simulink model "unidade3TestarBomba"  (R2015b)
settings: Solver=ode1  StartTime=0.0  StopTime=inf  FixedStep=0.002  RelTol=1e-3
PostLoadFcn:
  | qc_set_target_type(getConfigSet(bdroot, 'QUARC Default Target Configuration'));
undefined symbols (not defined in the file or in its folder): HIL
libraries: quarc_library x3
settings Model: SimulationMode=external  ExtModeTrigDuration=30000  Creator=MLevis  LastModifiedBy=UFRN
settings SolverCC: PositivePriorityOrder=on
settings DataIOCC: SaveFormat=Array  SignalLoggingSaveFormat=ModelDataLogs
settings OptimizationCC: ExpressionDepthLimit=2147483647  InitFltsAndDblsToZero=on
settings DebuggingCC: SaveWithParameterizedLinksMsg=none  UnderspecifiedInitializationDetection=Classic  MergeDetectMultiDrivingBlocksExec=none  SolverPrmCheckMsg=warning  MultiTaskDSMMsg=warning  MultiTaskCondExecSysMsg=none  FcnCallInpInsideContextMsg=UseLocalSettings  StateNameClashWarn=warning
settings HardwareCC: ProdBitPerPointer=32  ProdLargestAtomicFloat=None  ProdIntDivRoundTo=Undefined  ProdEndianess=Unspecified  ProdWordSize=32  ProdHWDeviceType=32-bit Generic
settings RTWCC: SystemTargetFile=quarc_win64.tlc  TemplateMakefile=quarc_default_tmf  Description=QUARC Win64 Target
settings GRTTargetCC: ParMdlRefBuildCompliant=off  CompOptLevelCompliant=off  GeneratePreprocessorConditionals=Disable all  CombineOutputUpdateFcns=off  MatFileLogging=off  GRTInterface=on  UseToolchainInfoCompliant=off  ExtMode=on  ExtModeMexFile=quarc_comm
settings ConfigComp: CovModelRefEnable=Off

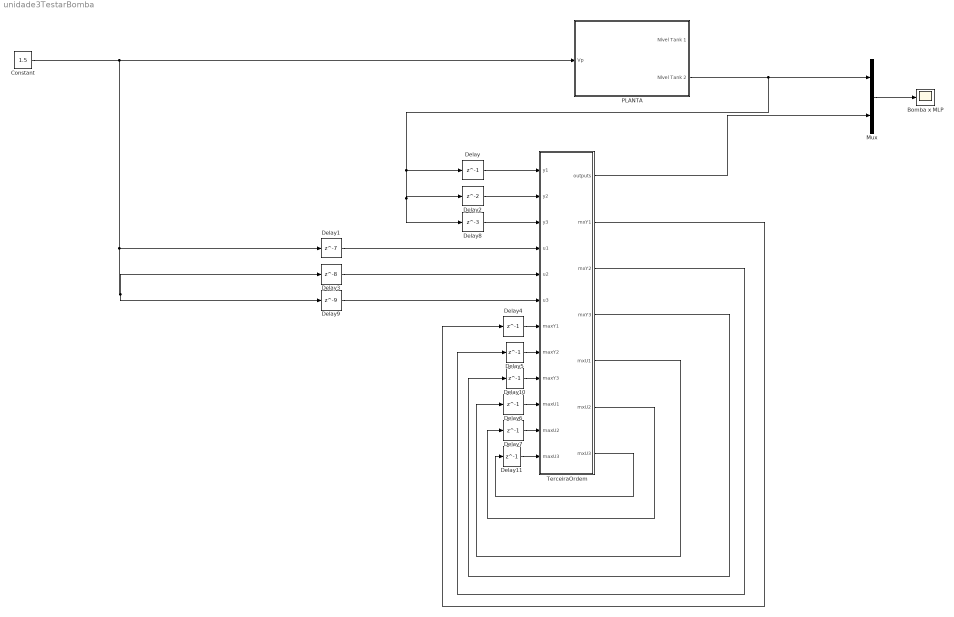
== system unidade3TestarBomba ==
  "Bomba x MLP " : Scope
  Constant : Constant  Value=1.5
  Delay{,4..7,10..11} (7 alike) : Delay  DelayLength=1  InitialCondition=0
  Delay1 : Delay  DelayLength=7  InitialCondition=0
  Delay2 : Delay  InitialCondition=0
  Delay3 : Delay  DelayLength=8  InitialCondition=0
  Delay8 : Delay  DelayLength=3  InitialCondition=0
  Delay9 : Delay  DelayLength=9  InitialCondition=0
  Mux : Mux  Inputs=2
  PLANTA : Subsystem
  "TerceiraOrdem " : MATLAB Function  TreatAsAtomicUnit=on
  wires:
  Mux/1 -> "Bomba x MLP "/1
  Delay/1 -> "TerceiraOrdem "/1(y1)
  Delay1/1 -> "TerceiraOrdem "/4(u1)
  Delay2/1 -> "TerceiraOrdem "/2(y2)
  Delay3/1 -> "TerceiraOrdem "/5(u2)
  PLANTA/2(Nível Tank 2) -> Delay2/1, Delay8/1, Delay/1, Mux/1
  Constant/1 -> Delay9/1, Delay3/1, Delay1/1, PLANTA/1(Vp)
  "TerceiraOrdem "/1(outputs) -> Mux/2
  "TerceiraOrdem "/2(mxY1) -> Delay4/1
  "TerceiraOrdem "/3(mxY2) -> Delay5/1
  Delay4/1 -> "TerceiraOrdem "/7(maxY1)
  Delay5/1 -> "TerceiraOrdem "/8(maxY2)
  Delay6/1 -> "TerceiraOrdem "/10(maxU1)
  Delay7/1 -> "TerceiraOrdem "/11(maxU2)
  Delay8/1 -> "TerceiraOrdem "/3(y3)
  Delay9/1 -> "TerceiraOrdem "/6(u3)
  Delay11/1 -> "TerceiraOrdem "/12(maxU3)
  Delay10/1 -> "TerceiraOrdem "/9(maxY3)
  "TerceiraOrdem "/4(mxY3) -> Delay10/1
  "TerceiraOrdem "/7(mxU3) -> Delay11/1
  "TerceiraOrdem "/6(mxU2) -> Delay7/1
  "TerceiraOrdem "/5(mxU1) -> Delay6/1

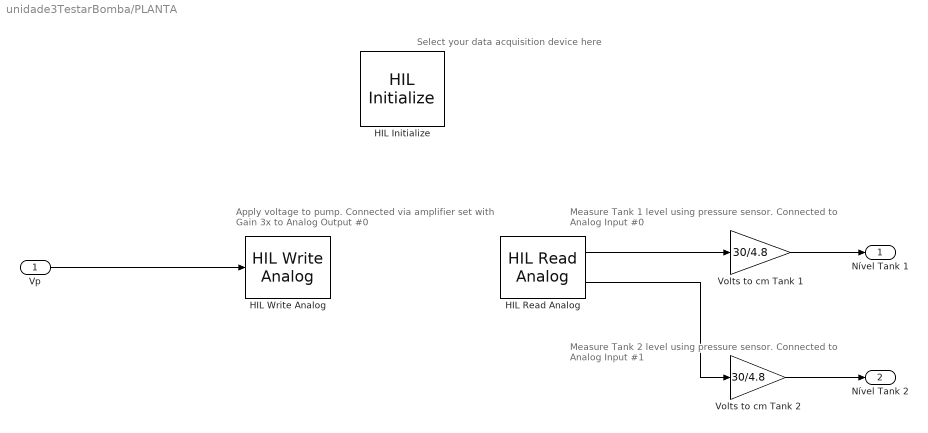
== system unidade3TestarBomba/PLANTA ==
  note: Select your data acquisition device here
  note: Apply voltage to pump.
      | Connected via amplifier set with Gain 3x
      | to  Analog Output #0
  note: Measure Tank 2 level using pressure sensor.
      | Connected to Analog Input #1
  note: Measure Tank 1 level using pressure sensor.
      | Connected to Analog Input #0
  Vp : Inport
  HIL Initialize : quarc_library/Data Acquisition/Generic/Configuration/HIL Initialize  object_name=HIL-1  board_type=q8_usb  board_number=0  board_options=update_rate=normal;decimation=1  exclusive=off  active=off  hardware_clocks=[0:2]  clock_modes=[]  initial_clock_frequencies=[]  set_clock_params_at_start=off  set_clock_params_at_switch_in=off  set_clock_frequencies_at_start=off  set_clock_frequencies_at_switch_in=off  analog_input_channels=[0:7]  analog_input_maximums=10  analog_input_minimums=-10  set_analog_input_params_at_start=on  set_analog_input_params_at_switch_in=off  analog_output_channels=[0:7]  analog_output_maximums=10  analog_output_minimums=-10  initial_analog_outputs=[0]  final_analog_outputs=[0]  watchdog_analog_outputs=0  set_analog_output_params_at_start=on  set_analog_output_params_at_switch_in=off  set_analog_outputs_at_start=on  set_analog_outputs_at_switch_in=off  set_analog_outputs_at_terminate=on  set_analog_outputs_at_switch_out=off  set_analog_outputs_on_watchdog=off  digital_input_channels=[]  digital_output_channels=[]  digital_output_configuration=[]  initial_digital_outputs=[1]  final_digital_outputs=[1]  watchdog_digital_outputs=[1]  set_digital_output_params_at_start=off  set_digital_output_params_at_switch_in=off  set_digital_outputs_at_start=on  set_digital_outputs_at_switch_in=off  set_digital_outputs_at_terminate=on  set_digital_outputs_at_switch_out=off  set_digital_outputs_on_watchdog=off  encoder_channels=[0:7]  quadrature=[4]  encoder_filter_frequency=[]  initial_encoder_counts=[0]  set_encoder_params_at_start=on  set_encoder_params_at_switch_in=off  set_encoder_counts_at_start=on  set_encoder_counts_at_switch_in=off  pwm_channels=[0:7]  pwm_modes=0  pwm_frequency=99.532799999999995e6/4095  pwm_configuration=[0]  pwm_alignment=[0]  pwm_polarity=[1]  pwm_leading_deadband=[0]  pwm_trailing_deadband=[0]  initial_pwm_outputs=[0]  final_pwm_outputs=[0]  watchdog_pwm_outputs=[0]  set_pwm_params_at_start=on  set_pwm_params_at_switch_in=off  set_pwm_outputs_at_start=on  set_pwm_outputs_at_switch_in=off  set_pwm_outputs_at_terminate=on  set_pwm_outputs_at_switch_out=off  set_pwm_outputs_on_watchdog=off  other_output_channels=[]  initial_other_outputs=[]  final_other_outputs=[]  watchdog_other_outputs=[]  set_other_outputs_at_start=off  set_other_outputs_at_switch_in=off  set_other_outputs_at_terminate=off  set_other_outputs_at_switch_out=off  set_other_outputs_on_watchdog=off
  HIL Read Analog : quarc_library/Data Acquisition/Generic/Immediate I//O/HIL Read Analog  object_name=HIL-1  channels=[0:1]  sample_time=qc_get_step_size  active=on  vector_output=off
  HIL Write Analog : quarc_library/Data Acquisition/Generic/Immediate I//O/HIL Write Analog  object_name=HIL-1  channels=0  sample_time=-1  active=off  vector_input=off
  "Volts to cm Tank 1 " : Gain  Gain=30/4.8
  Volts to cm Tank 2 : Gain  Gain=30/4.8
  Nível Tank 1 : Outport
  Nível Tank 2 : Outport  Port=2
  wires:
  HIL Read Analog/1 -> "Volts to cm Tank 1 "/1
  HIL Read Analog/2 -> Volts to cm Tank 2/1
  Vp/1 -> HIL Write Analog/1
  "Volts to cm Tank 1 "/1 -> Nível Tank 1/1
  Volts to cm Tank 2/1 -> Nível Tank 2/1

== matlab function unidade3TestarBomba/TerceiraOrdem  ==
  data: y1 input; y2 input; y3 input; u1 input; outputs output; u2 input; u3 input; maxY1 input; maxY2 input; maxY3 input; maxU1 input; maxU2 input; mxY1 output; mxY2 output; mxY3 output; mxU1 output; mxU2 output; maxU3 input; mxU3 output
%% Ordem 3, Atraso 7
function [outputs,mxY1,mxY2,mxY3,mxU1,mxU2,mxU3] = EvaluateNetworkForSimulink(y1,y2,y3,u1,u2,u3,maxY1,maxY2,maxY3,maxU1,maxU2,maxU3)
%nbrOfLayers = length(nce);
PesosIn=[-0.0001    0.1868    0.2669    0.6229   -0.0869   -0.3360    0.5296    0.1765   -0.6396   -0.3845    0.1475    0.4356   -0.7523   -0.9999    0.7666   -0.7905;
   -0.0045   -0.9917    0.9704    0.5207    0.3732   -0.9040    0.3163   -0.6453    0.9121   -0.5066    1.0073    0.5780   -0.5972    0.5690   -0.2224   -0.2149;
   -0.0045    0.7956   -0.1117    0.9859   -0.8032   -0.8241    0.7744    0.9662    0.9786    0.3330    0.4970    0.2092   -0.4549    0.4778   -0.5242   -0.4115;
   -0.0045   -0.6679   -0.6808    0.4005    0.2551    0.6710    0.9458    0.1064    1.0170    0.6773    0.6005    1.0138    0.7089    1.0327   -0.6141   -0.0496;
   -0.0030   -0.9360    0.8276    0.1029    0.8001    0.6065    0.6205    0.4331   -0.1274    0.6513    0.3400   -0.5211   -0.0314    0.4916    0.6307    0.5400;
   -0.0030    0.7298    0.3081   -0.5846   -0.7400    0.7848    0.2346   -0.2358   -0.5107    0.4968   -0.4603    0.0807   -0.3254   -0.4689   -0.5965    0.9197;
   -0.0027   -0.9687   -0.1611    0.7042   -0.4113    0.0497   -0.3168    0.3694   -0.7001    0.8131   -0.1828    0.9144   -0.7451   -0.3586   -0.9271    0.6353];



PesosEsc=[-0.1139;
   -0.2709;
   -0.0339;
    0.1325;
   -0.1239;
   -0.1974;
    0.1379;
    0.0226;
    0.4551;
    0.0675;
    0.2632;
    0.1527;
   -0.0971;
    0.4322;
   -0.4362;
   -0.0359];



PesosOut=1;



maxY1=max(maxY1,y1);
maxY2=max(maxY2,y2);
maxY3=max(maxY3,y3);
maxU1=max(maxU1,u1);
maxU2=max(maxU2,u2);
maxU3=max(maxU3,u3);

y1=y1./maxY1;
y2=y2./maxY2;
y3=y3./maxY3;
u1=u1./maxU1;
u2=u2./maxU2;
u3=u3./maxU3;

Sample=[y1 y2 y3 u1 u2 u3];
Sample = [ones(length(Sample(:,1)),1) Sample];

NodeIn = Sample;

NodeIn = NodeIn*PesosIn;



NodeIn = FuncaoAtivacao(NodeIn,'LOGSIGMOIDE');

NodeHid=NodeIn;


NodeHid = NodeHid*PesosEsc;

NodeHid = FuncaoAtivacao(NodeHid,'LOGSIGMOIDE');


NodeOut=NodeHid;
NodeOut = NodeOut*PesosOut;

outputs=NodeOut.*max(maxY1,max(maxY2,max( maxY3,max( maxU3,max(maxU1,maxU2) ) )  ));

mxY1=maxY1;
mxY2=maxY2;
mxY3=maxY3;
mxU1=maxU1;
mxU2=maxU2;
mxU3=maxU3;
end
